simulink model "LKA_Lenkung_CarMaker_DSR_kombiniert"  (Simulink 8.9)
settings: Solver=ode23  StartTime=0.0  StopTime=tend  FixedStep=0.01  RelTol=1e-3  EnableMultiTasking=on
undefined symbols (not defined in the file or in its folder): contr, pin
libraries: library x7, simulink x3
settings Model: Creator=Georg  LastModifiedBy=Georg
settings OptimizationCC: ExpressionDepthLimit=2147483647
settings DebuggingCC: SolverPrmCheckMsg=warning

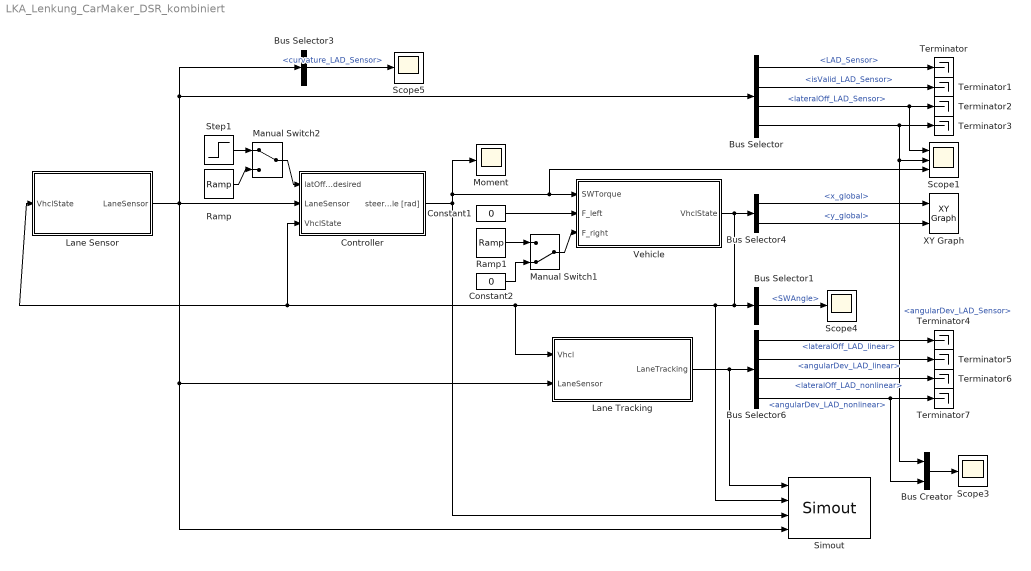
== system LKA_Lenkung_CarMaker_DSR_kombiniert ==
  Bus Creator : BusCreator  Inputs=2
  Bus Selector : BusSelector  OutputSignals=LAD_Sensor,isValid_LAD_Sensor,lateralOff_LAD_Sensor,angularDev_LAD_Sensor
  Bus Selector1 : BusSelector  OutputSignals=SWAngle
  Bus Selector3 : BusSelector  OutputSignals=curvature_LAD_Sensor
  Bus Selector4 : BusSelector  OutputSignals=x_global,y_global
  Bus Selector6 : BusSelector  OutputSignals=lateralOff_LAD_linear,angularDev_LAD_linear,lateralOff_LAD_nonlinear,angularDev_LAD_nonlinear
  Constant1 : Constant  Value=0
  Constant2 : Constant  Value=0
  Controller : Subsystem
  Lane Sensor : Subsystem
  Lane Tracking : Subsystem
  Manual Switch1 : ManualSwitch  CurrentSetting=0
  Manual Switch2 : ManualSwitch
  Moment : Scope
  Ramp : simulink/Sources/Ramp  slope=1  start=10  X0=0
  Ramp1 : simulink/Sources/Ramp  slope=1  start=10  X0=0
  Scope1 : Scope  NumInputPorts=3
  Scope3 : Scope
  Scope4 : Scope
  Scope5 : Scope
  Simout : library/Misc/Simout
  Step1 : Step  Time=10  After=0  SampleTime=0
  Terminator{,1..7} (8 alike) : Terminator
  Vehicle : Subsystem
  XY Graph : simulink/Sinks/XY Graph  xmin=-50  xmax=700  ymin=-10  ymax=600  st=-1
  wires:
  Bus Selector4/1 -> XY Graph/1  "<x_global>"
  Bus Selector4/2 -> XY Graph/2  "<y_global>"
  Bus Creator/1 -> Scope3/1
  Ramp1/1 -> Manual Switch1/1
  Constant2/1 -> Manual Switch1/2
  Manual Switch1/1 -> Vehicle/3(F_right)
  Bus Selector3/1 -> Scope5/1  "<curvature_LAD_Sensor>"
  Manual Switch2/1 -> Controller/1(latOff_LAD_desired)
  Constant1/1 -> Vehicle/2(F_left)
  Step1/1 -> Manual Switch2/1
  Ramp/1 -> Manual Switch2/2
  Controller/1(steerAngle [rad]) -> Vehicle/1(SWTorque), Scope1/3, Moment/1, Simout/3
  Vehicle/1(VhclState) -> Bus Selector4/1, Bus Selector1/1, Lane Tracking/1(Vhcl), Controller/3(VhclState), Lane Sensor/1(VhclState), Simout/2
  Lane Sensor/1(LaneSensor) -> Controller/2(LaneSensor), Bus Selector3/1, Bus Selector/1, Lane Tracking/2(LaneSensor), Simout/4
  Bus Selector6/1 -> Terminator4/1  "<lateralOff_LAD_linear>"
  Bus Selector6/2 -> Terminator5/1  "<angularDev_LAD_linear>"
  Bus Selector6/3 -> Terminator6/1  "<lateralOff_LAD_nonlinear>"
  Bus Selector6/4 -> Terminator7/1, Bus Creator/2  "<angularDev_LAD_nonlinear>"
  Bus Selector/1 -> Terminator/1  "<LAD_Sensor>"
  Bus Selector/2 -> Terminator1/1  "<isValid_LAD_Sensor>"
  Bus Selector/3 -> Terminator2/1, Scope1/1  "<lateralOff_LAD_Sensor>"
  Bus Selector/4 -> Terminator3/1, Scope1/2, Bus Creator/1  "<angularDev_LAD_Sensor>"
  Lane Tracking/1(LaneTracking) -> Bus Selector6/1, Simout/1
  Bus Selector1/1 -> Scope4/1  "<SWAngle>"

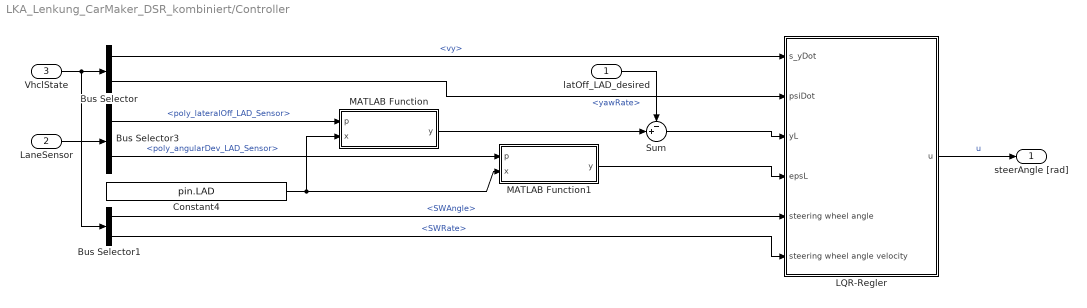
== system LKA_Lenkung_CarMaker_DSR_kombiniert/Controller ==
  latOff_LAD_desired : Inport
  LaneSensor : Inport  Port=2
  VhclState : Inport  Port=3
  Bus Selector : BusSelector  OutputSignals=vy,yawRate
  Bus Selector1 : BusSelector  OutputSignals=SWAngle,SWRate
  Bus Selector3 : BusSelector  OutputSignals=poly_lateralOff_LAD_Sensor,poly_angularDev_LAD_Sensor
  Constant4 : Constant  Value=pin.LAD
  LQR-Regler : Subsystem
  MATLAB Function : MATLAB Function  TreatAsAtomicUnit=on
  MATLAB Function1 : MATLAB Function  TreatAsAtomicUnit=on
  Sum : Sum  Inputs=-+|
  steerAngle [rad] : Outport
  wires:
  MATLAB Function1/1(y) -> LQR-Regler/4(epsL)
  Constant4/1 -> MATLAB Function1/2(x), MATLAB Function/2(x)
  LaneSensor/1 -> Bus Selector3/1
  LQR-Regler/1(u) -> steerAngle [rad]/1  "u"
  Bus Selector3/1 -> MATLAB Function/1(p)  "<poly_lateralOff_LAD_Sensor>"
  Bus Selector3/2 -> MATLAB Function1/1(p)  "<poly_angularDev_LAD_Sensor>"
  VhclState/1 -> Bus Selector/1, Bus Selector1/1
  Bus Selector/1 -> LQR-Regler/1(s_yDot)  "<vy>"
  Bus Selector/2 -> LQR-Regler/2(psiDot)  "<yawRate>"
  Bus Selector1/1 -> LQR-Regler/5(steering wheel angle)  "<SWAngle>"
  Bus Selector1/2 -> LQR-Regler/6(steering wheel angle velocity)  "<SWRate>"
  MATLAB Function/1(y) -> Sum/2
  Sum/1 -> LQR-Regler/3(yL)
  latOff_LAD_desired/1 -> Sum/1

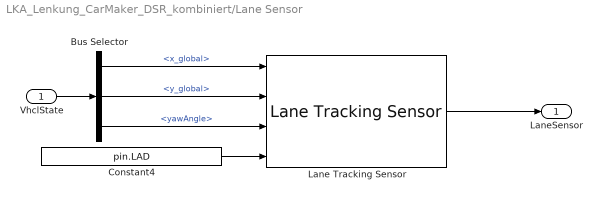
== system LKA_Lenkung_CarMaker_DSR_kombiniert/Lane Sensor ==
  VhclState : Inport
  Bus Selector : BusSelector  OutputSignals=x_global,y_global,yawAngle
  Constant4 : Constant  Value=pin.LAD
  Lane Tracking Sensor : library/Lane Tracking/Lane Tracking Sensor
  LaneSensor : Outport
  wires:
  Lane Tracking Sensor/1 -> LaneSensor/1
  VhclState/1 -> Bus Selector/1
  Bus Selector/1 -> Lane Tracking Sensor/1  "<x_global>"
  Bus Selector/2 -> Lane Tracking Sensor/2  "<y_global>"
  Bus Selector/3 -> Lane Tracking Sensor/3  "<yawAngle>"
  Constant4/1 -> Lane Tracking Sensor/4

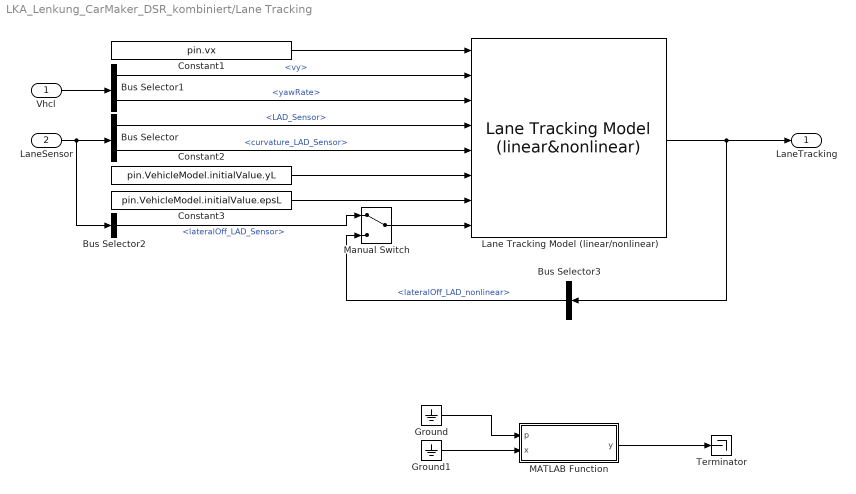
== system LKA_Lenkung_CarMaker_DSR_kombiniert/Lane Tracking ==
  Vhcl : Inport
  LaneSensor : Inport  Port=2
  Bus Selector : BusSelector  OutputSignals=LAD_Sensor,curvature_LAD_Sensor
  Bus Selector1 : BusSelector  OutputSignals=vy,yawRate
  Bus Selector2 : BusSelector  OutputSignals=lateralOff_LAD_Sensor
  Bus Selector3 : BusSelector  OutputSignals=lateralOff_LAD_nonlinear
  Constant1 : Constant  Value=pin.vx
  Constant2 : Constant  Value=pin.VehicleModel.initialValue.yL
  Constant3 : Constant  Value=pin.VehicleModel.initialValue.epsL
  Ground : Ground
  Ground1 : Ground
  Lane Tracking Model (linear/nonlinear) : library/Lane Tracking/Lane Tracking Model (linear&nonlinear)
  MATLAB Function : MATLAB Function  TreatAsAtomicUnit=on
  Manual Switch : ManualSwitch
  Terminator : Terminator
  LaneTracking : Outport
  wires:
  LaneSensor/1 -> Bus Selector/1, Bus Selector2/1
  Constant2/1 -> Lane Tracking Model (linear/nonlinear)/6
  Constant3/1 -> Lane Tracking Model (linear/nonlinear)/7
  Vhcl/1 -> Bus Selector1/1
  Constant1/1 -> Lane Tracking Model (linear/nonlinear)/1
  Bus Selector1/1 -> Lane Tracking Model (linear/nonlinear)/2  "<vy>"
  Bus Selector1/2 -> Lane Tracking Model (linear/nonlinear)/3  "<yawRate>"
  Bus Selector/1 -> Lane Tracking Model (linear/nonlinear)/4  "<LAD_Sensor>"
  Bus Selector/2 -> Lane Tracking Model (linear/nonlinear)/5  "<curvature_LAD_Sensor>"
  Bus Selector3/1 -> Manual Switch/2  "<lateralOff_LAD_nonlinear>"
  Bus Selector2/1 -> Manual Switch/1  "<lateralOff_LAD_Sensor>"
  Manual Switch/1 -> Lane Tracking Model (linear/nonlinear)/8
  Lane Tracking Model (linear/nonlinear)/1 -> Bus Selector3/1, LaneTracking/1
  Ground/1 -> MATLAB Function/1(p)
  Ground1/1 -> MATLAB Function/2(x)
  MATLAB Function/1(y) -> Terminator/1

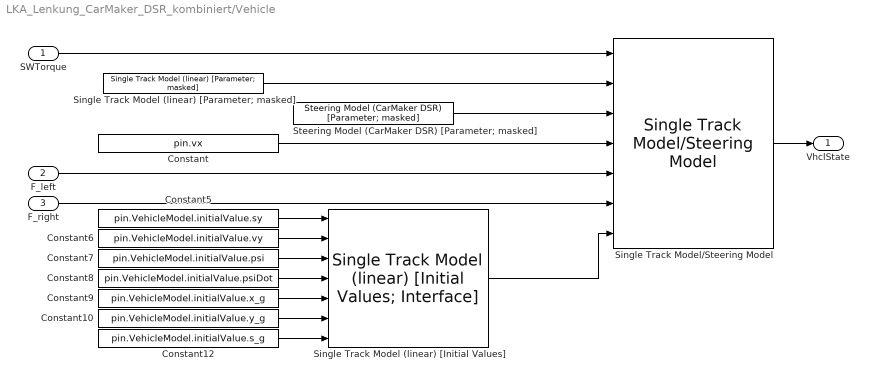
== system LKA_Lenkung_CarMaker_DSR_kombiniert/Vehicle ==
  SWTorque : Inport
  F_left : Inport  Port=2
  F_right : Inport  Port=3
  Constant : Constant  Value=pin.vx
  Constant10 : Constant  Value=pin.VehicleModel.initialValue.y_g
  Constant12 : Constant  Value=pin.VehicleModel.initialValue.s_g
  Constant5 : Constant  Value=pin.VehicleModel.initialValue.sy
  Constant6 : Constant  Value=pin.VehicleModel.initialValue.vy
  Constant7 : Constant  Value=pin.VehicleModel.initialValue.psi
  Constant8 : Constant  Value=pin.VehicleModel.initialValue.psiDot
  Constant9 : Constant  Value=pin.VehicleModel.initialValue.x_g
  Single Track Model (linear) [Initial Values] : library/Vehicle Models ext./Single Track Model (linear) [Initial Values; Interface]
  Single Track Model (linear) [Parameter; masked] : library/Vehicle Models ext./Single Track Model (linear) [Parameter; masked]  cs_front=pin.VehicleModel.parameter.csv  cs_rear=pin.VehicleModel.parameter.csh  l_front=pin.VehicleModel.parameter.lv  l_rear=pin.VehicleModel.parameter.lh  m=pin.VehicleModel.parameter.m  Izz=pin.VehicleModel.parameter.Iz
  Single Track Model/Steering Model : library/Vehicle Models ext./Single Track Model//Steering Model
  Steering Model (CarMaker DSR) [Parameter; masked] : library/Vehicle Models ext./Steering Model (CarMaker DSR) [Parameter; masked]  d_rot=pin.SteeringModel.parameter.drot  d_rack=pin.SteeringModel.parameter.drack  i_HR=pin.SteeringModel.parameter.iHR  I_rot=pin.SteeringModel.parameter.J  m_left=pin.SteeringModel.parameter.mL  m_right=pin.SteeringModel.parameter.mR  m_rack=pin.SteeringModel.parameter.mr  V=pin.SteeringModel.parameter.V  alpha=pin.SteeringModel.parameter.alph
  VhclState : Outport
  wires:
  Steering Model (CarMaker DSR) [Parameter; masked]/1 -> Single Track Model/Steering Model/3
  Constant/1 -> Single Track Model/Steering Model/4
  SWTorque/1 -> Single Track Model/Steering Model/1
  Single Track Model (linear) [Parameter; masked]/1 -> Single Track Model/Steering Model/2
  Constant5/1 -> Single Track Model (linear) [Initial Values]/1
  Constant6/1 -> Single Track Model (linear) [Initial Values]/2
  Constant7/1 -> Single Track Model (linear) [Initial Values]/3
  Constant8/1 -> Single Track Model (linear) [Initial Values]/4
  Constant9/1 -> Single Track Model (linear) [Initial Values]/5
  Constant10/1 -> Single Track Model (linear) [Initial Values]/6
  Constant12/1 -> Single Track Model (linear) [Initial Values]/7
  Single Track Model (linear) [Initial Values]/1 -> Single Track Model/Steering Model/7
  F_left/1 -> Single Track Model/Steering Model/5
  F_right/1 -> Single Track Model/Steering Model/6
  Single Track Model/Steering Model/1 -> VhclState/1

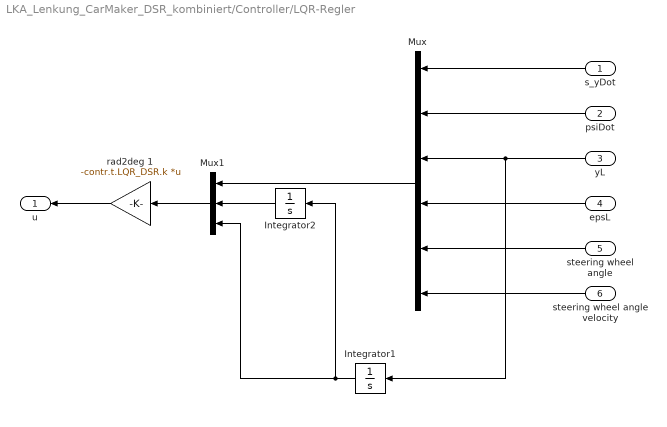
== system LKA_Lenkung_CarMaker_DSR_kombiniert/Controller/LQR-Regler ==
  s_yDot : Inport
  psiDot : Inport  Port=2
  yL : Inport  Port=3
  epsL : Inport  Port=4
  steering wheel angle : Inport  Port=5
  steering wheel angle velocity : Inport  Port=6
  Integrator1 : Integrator
  Integrator2 : Integrator
  Mux : Mux  Inputs=6
  Mux1 : Mux  Inputs=3
  rad2deg 1 : Gain  Gain=-contr.t.LQR_DSR.k  Multiplication=Matrix(K*u) (u vector)
  u : Outport
  wires:
  Mux/1 -> Mux1/1
  Mux1/1 -> rad2deg 1/1
  yL/1 -> Mux/3, Integrator1/1
  s_yDot/1 -> Mux/1
  psiDot/1 -> Mux/2
  rad2deg 1/1 -> u/1
  epsL/1 -> Mux/4
  steering wheel angle/1 -> Mux/5
  steering wheel angle velocity/1 -> Mux/6
  Integrator2/1 -> Mux1/2
  Integrator1/1 -> Integrator2/1, Mux1/3

== matlab function Controller/MATLAB Function ==
  data: p input double; y output double; x input double
function y = polyVal(p,x)
%#codegen

y = polyval(p,x);

== matlab function Controller/MATLAB Function1 ==
  data: p input double; y output double; x input double
function y = polyVal(p,x)
%#codegen

y = polyval(p,x);

== matlab function Lane Tracking/MATLAB Function ==
  data: p input double; y output double; x input double
function y = polyVal(p,x)
%#codegen

y = polyval(p,x);
